simulink model "simulacion_control"  (R2021a)
settings: Solver=ode4  StartTime=0.0  StopTime=50  FixedStep=0.002  RelTol=1e-3
settings Model: Creator=amddy  LastModifiedBy=Jorge_Sarmiento
settings DataIOCC: SaveFormat=Array  SignalLogging=off  DSMLogging=off  TimeSaveName=time_simulink  OutputSaveName=y_simulink  ReturnWorkspaceOutputsName=simulink

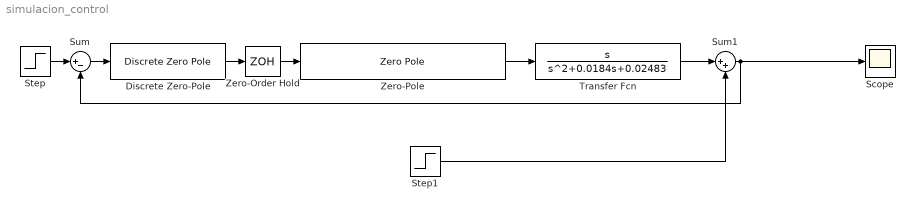
== system simulacion_control ==
  Discrete Zero-Pole : DiscreteZeroPole  Zeros=[1 1]  Poles=[1 -1]  Gain=100.03  SampleTime=0.02
  Scope : Scope
  Step : Step  Time=0  After=0  SampleTime=0.02
  Step1 : Step  Time=0.5  After=-22  SampleTime=0
  Sum : Sum  Inputs=|+-
  Sum1 : Sum  Inputs=|++
  Transfer Fcn : TransferFcn  Numerator=[1 0]  Denominator=[1 0.0184 0.02483]
  Zero-Order Hold : ZeroOrderHold  SampleTime=0.02
  Zero-Pole : ZeroPole  Zeros=[-0.0543 -0.0047]  Poles=[-0.5809 -0.065]  Gain=0.6942
  wires:
  Step/1 -> Sum/1
  Sum/1 -> Discrete Zero-Pole/1
  Discrete Zero-Pole/1 -> Zero-Order Hold/1
  Zero-Order Hold/1 -> Zero-Pole/1
  Sum1/1 -> Sum/2, Scope/1
  Transfer Fcn/1 -> Sum1/1
  Zero-Pole/1 -> Transfer Fcn/1
  Step1/1 -> Sum1/2
